simulink model "slx"  (R2014a)
settings: Solver=ode45  StartTime=0.0  StopTime=10.0  RelTol=1e-3
libraries: fl_lib x4
settings Model: Creator=UTILISATEUR  LastModifiedBy=UTILISATEUR

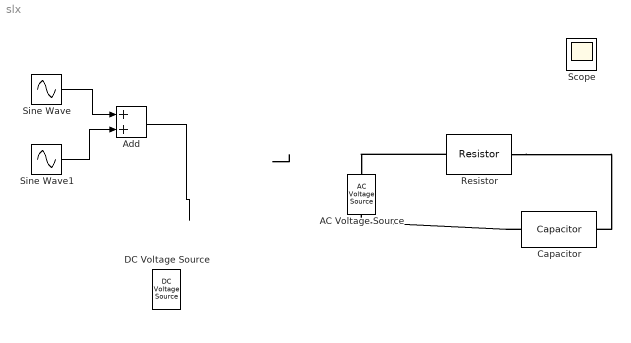
== system slx ==
  AC Voltage Source : fl_lib/Electrical/Electrical Sources/AC Voltage Source  amp=10 V  shift=0 deg  frequency=1000 Hz  omega=0 rad/s
  Add : Sum
  Capacitor : fl_lib/Electrical/Electrical Elements/Capacitor  c=100 nF  r=1e-6 Ohm  g=0 1/Ohm  i_specify=off  i_priority=High  i=0 A  v_specify=off  v_priority=High  v=0 V  vc_specify=off  vc_priority=High  vc=0 V
  DC Voltage Source : fl_lib/Electrical/Electrical Sources/DC Voltage Source  v0=1 V
  Resistor : fl_lib/Electrical/Electrical Elements/Resistor  R=1 kOhm  i_specify=off  i_priority=High  i=0 A  v_specify=off  v_priority=High  v=0 V
  Scope : Scope
      settings: TimeRange=10
  Sine Wave : Sin  Amplitude=10  Frequency=1000  SampleTime=0
  Sine Wave1 : Sin  Amplitude=10  Frequency=10  SampleTime=0
  wires:
  Sine Wave/1 -> Add/1
  Sine Wave1/1 -> Add/2
  Add/1 -> ?
  ? -> Scope/1
  connections:
  ?
  Resistor/RConn1 -- Capacitor/RConn1
  Capacitor/LConn1 -- AC Voltage Source/RConn1
  Resistor/LConn1 -- AC Voltage Source/LConn1
